simulink model "dsmDemo"  (R2017a)
settings: Solver=VariableStepAuto  StartTime=0.0  StopTime=10000  RelTol=1e-3
undefined symbols (not defined in the file or in its folder): sigbuilder_block
settings Model: Creator=XJ  LastModifiedBy=XJ

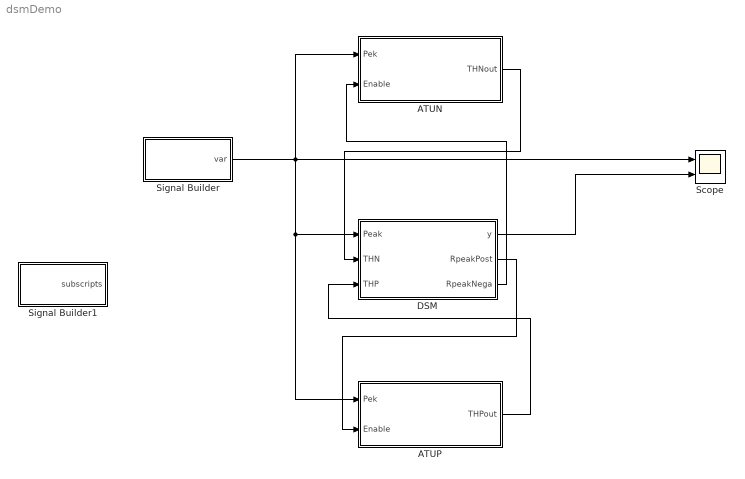
== system dsmDemo ==
  ATUN : MATLAB Function  TreatAsAtomicUnit=on
  ATUP : MATLAB Function  TreatAsAtomicUnit=on
  DSM : Stateflow chart  TreatAsAtomicUnit=on
  Scope : Scope  NumInputPorts=2
  Signal Builder : Subsystem  Tag=STV Subsys  LoadFcn=sigbuilder_block('load',[293.25 110.25 519 399.75 ]);  StartFcn=sigbuilder_block('start');  StopFcn=sigbuilder_block('stop');  ClipboardFcn=sigbuilder_block('clipboard');  mask(Sigbuilder block){tuvar=[0:10]}
      mask help: Simulink:masks:SigbuilderBlock_MD
      mask init:
      | if ~strcmp(get_param(bdroot(gcbh),'SimulationStatus'),'stopped') tuvar = sigbuilder_block('maskInit'); end
      settings: CopyFcn=sigbuilder_block('copy');  DeleteFcn=sigbuilder_block('delete');  ModelCloseFcn=sigbuilder_block('modelClose');  PreSaveFcn=sigbuilder_block('preSave');  PauseFcn=sigbuilder_block('pause');  ContinueFcn=sigbuilder_block('continue');  NameChangeFcn=sigbuilder_block('namechange');  OpenFcn=sigbuilder_block('open',[253.5 32.25 519 399.75 ]);  CloseFcn=sigbuilder_block('close');
      mask Display: plot(0, 0, 100, 100,[2, 2, 32, 32, 2], [68, 8, 8, 68, 68],[32, 2], [38, 38], [32, 19, 2],[53, 60, 44], [32, 17, 17, 2],[16, 16, 31, 31]);txt = getActiveGroup(gcbh);text(2, 100, txt,'verticalAlignment', 'top');
  Signal Builder1 : Subsystem  Tag=STV Subsys  LoadFcn=sigbuilder_block('load');  StartFcn=sigbuilder_block('start');  StopFcn=sigbuilder_block('stop');  ClipboardFcn=sigbuilder_block('clipboard');  mask(Sigbuilder block){tuvar=[0:10]}
      mask help: Simulink:masks:SigbuilderBlock_MD
      mask init:
      | if ~strcmp(get_param(bdroot(gcbh),'SimulationStatus'),'stopped') tuvar = sigbuilder_block('maskInit'); end
      settings: CopyFcn=sigbuilder_block('copy');  DeleteFcn=sigbuilder_block('delete');  ModelCloseFcn=sigbuilder_block('modelClose');  PreSaveFcn=sigbuilder_block('preSave');  PauseFcn=sigbuilder_block('pause');  ContinueFcn=sigbuilder_block('continue');  NameChangeFcn=sigbuilder_block('namechange');  OpenFcn=sigbuilder_block('open',[364.5 63.75 550.5 399.75 ]);  CloseFcn=sigbuilder_block('close');
      mask Display: plot(0, 0, 100, 100,[2, 2, 32, 32, 2], [68, 8, 8, 68, 68],[32, 2], [38, 38], [32, 19, 2],[53, 60, 44], [32, 17, 17, 2],[16, 16, 31, 31]);txt = getActiveGroup(gcbh);text(2, 100, txt,'verticalAlignment', 'top');
  wires:
  Signal Builder/1(var) -> ATUP/1(Pek), DSM/1(Peak), ATUN/1(Pek), Scope/1
  DSM/1(y) -> Scope/2
  DSM/2(RpeakPost) -> ATUP/2(Enable)
  ATUP/1(THPout) -> DSM/3(THP)
  DSM/3(RpeakNega) -> ATUN/2(Enable)
  ATUN/1(THNout) -> DSM/2(THN)

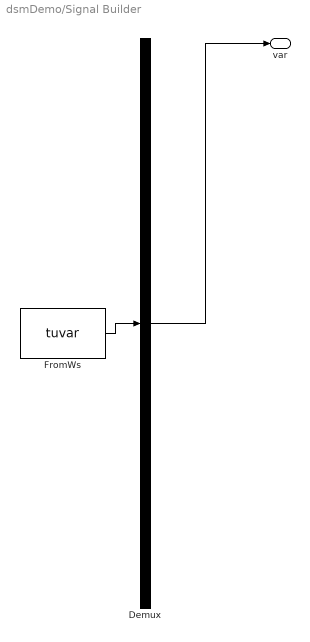
== system dsmDemo/Signal Builder ==
  Demux : Demux  Tag=STV Demux  Outputs=1
  FromWs : FromWorkspace  Tag=STV FromWs  VariableName=tuvar  SampleTime=0
      SigBuilderData=|
      | common.afterFinalStr = 'Extrapolate'
      | common.sampleTime = 0
      | dataSet.timeRange = [1 10000]
      | dataSet.name = 'Imported_Group 1'
      | sbobj.Groups.Name = 'Imported_Group 1'
      | sbobj.Groups.Signals.Name = 'var'
      | sbobj.Groups.Signals.XData = [1 2 3 4 5 6 7 8 9 10 11 12 ... (10000 elements, 1x10000)]
      | sbobj.Groups.Signals.YData = [0 0 0 0 0 0 0 0.0025 0 0 0 0 ... (10000 elements, 1x10000)]
      | sbobj.Groups.TimeRange = [1 10000]
  var : Outport  Tag=STV Outport
  wires:
  Demux/1 -> var/1
  FromWs/1 -> Demux/1

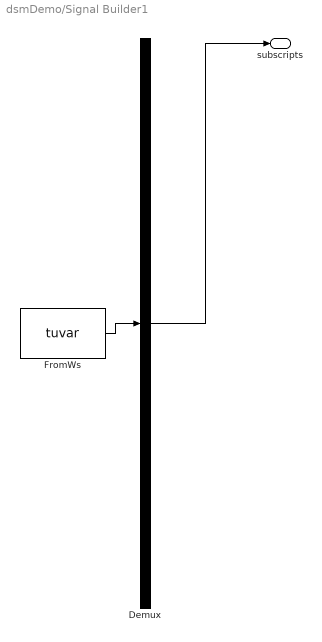
== system dsmDemo/Signal Builder1 ==
  Demux : Demux  Tag=STV Demux  Outputs=1
  FromWs : FromWorkspace  Tag=STV FromWs  VariableName=tuvar  SampleTime=0
      SigBuilderData=|
      | common.afterFinalStr = 'Extrapolate'
      | common.sampleTime = 0
      | dataSet.timeRange = [1 10000]
      | dataSet.name = 'Imported_Group 1'
      | sbobj.Groups.Name = 'Imported_Group 1'
      | sbobj.Groups.Signals.Name = 'subscripts'
      | sbobj.Groups.Signals.XData = [1 2 3 4 5 6 7 8 9 10 11 12 ... (10000 elements, 1x10000)]
      | sbobj.Groups.Signals.YData = [1 2 3 4 5 6 7 8 9 10 11 12 ... (10000 elements, 1x10000)]
      | sbobj.Groups.TimeRange = [1 10000]
  subscripts : Outport  Tag=STV Outport
  wires:
  Demux/1 -> subscripts/1
  FromWs/1 -> Demux/1

== matlab function dsmDemo/ATUN ==
  data: Pek input; THNout output; Enable input
function THNout = ma(Pek,Enable)
% Declare one persistent vectors
persistent sum cnt alpha temp
% Initialize the variables
if isempty(sum)
    sum = zeros(1,8);
    cnt = int32(0);
    alpha = 1;
    temp = -0.3;
end
% Compute the accumulated sum and the number of values so far.
if Enable ==1 
    cnt = cnt + 1;
    switch cnt
        case (cnt<8)
          sum(cnt) = Pek;
          THNout = -0.3;
        case (cnt == 8)
          sum(cnt) = Pek;
          THNout = alpha * mean(sum);
        otherwise
          sum(mod(cnt,8)) = Pek;
          THNout = alpha * mean(sum);
    end
    temp = THNout;
else
    THNout = temp; 
end

== stateflow chart dsmDemo/DSM ==
  state Ready
    entry: y=0;
  state P_Peak1
    entry:RpeakPost=1;
    during: RpeakPost=0,CountP = CountP +1;
  state N_Peak1
    entry:RpeakNega = 1;
    during: RpeakPost = 0,CountN = CountN + 1;
  state N_Peak2
  state P_Peak2
  state Peak_Pair
    entry: y=1;
    during: y=0,CountPair = CountPair + 1;
  (default) -> Ready
  Ready -> Ready [order 2] : [(Peak<THP)&&(Peak>THN)]
  Peak_Pair -> Ready : [CountPair>=t_h2]{CountPair = 0}
  P_Peak1 -> Ready [order 1] : [CountP>=t_h1]{CountP = 0}
  N_Peak1 -> Ready [order 1] : [CountN>=t_h1]{CountN = 0}
  Ready -> P_Peak1 [order 3] : [Peak>THP]
  Ready -> N_Peak1 [order 1] : [Peak<THN]
  P_Peak1 -> N_Peak2 [order 2] : [Peak<THN]
  N_Peak1 -> P_Peak2 [order 2] : [Peak>THP]
  N_Peak2 -> Peak_Pair
  P_Peak2 -> Peak_Pair
  data: Peak input; CountN local =0; t_h1 constant double =54; y output; t_h2 constant double =50; CountP local =0; CountPair local =0; THN input double =-0.3; THP input double =0.3; RpeakPost output; RpeakNega output

== matlab function dsmDemo/ATUP ==
  data: Pek input; THPout output; Enable input
function THPout = ma(Pek,Enable)
% Declare one persistent vectors
persistent sum cnt alpha temp
% Initialize the variables
if isempty(sum)
    sum = zeros(1,8);
    cnt = int32(0);
    alpha = 1;
    temp = 0.3;
end
% Compute the accumulated sum and the number of values so far.
if Enable ==1 
    cnt = cnt + 1;
    switch cnt
        case (cnt<8)
          sum(cnt) = Pek;
          THPout = 0.3;
        case (cnt == 8)
          sum(cnt) = Pek;
          THPout = alpha * mean(sum);
        otherwise
          sum(mod(cnt,8)) = Pek;
          THPout = alpha * mean(sum);
    end
    temp = THPout;
else
    THPout = temp; 
end
